simulink model "PWM_Test"  (Simulink 7.7)
settings: Solver=ode4  StartTime=0.0  StopTime=inf  FixedStep=sample_time  RelTol=1e-3
InitFcn:
  | sample_time=0.005;%0.004;%0.0025;%0.02;
  | DeltaT = 0.02;
  | g = 9.81;
  | H0 = g%0.3165;
  | Kl = 1;
  | 
  | Omega_r = 1.6;%for Horizontal reference
  | Zeta_r = 1; %for Horizontal reference
  | Omega = 1.8;%for Horizontal Control
  | Zeta = 0.5;    %for Horizontal Control
  | 
  | Omega_h_r = 2.5; %for vertical reference
  | Zeta_h_r = 0.8;  %for vertical reference
  | Omega_h = 2.7;    %for vertical control
  | Zeta_h = 0.8;         %for vertical control
  | PI=pi;
  | 
  | Mass = 1.15;
  | Acc_Max = 4;
  | Acc_Max_h = 4;
  | 
  | Max_RP = 60;
  | 
  | % for NN
  | n = 5;
  | r = 3;
  | n2 = 5;
  | NN_ST = 0.02;
  | 
  | GAMA_V = 6;
  | gama_V_e = 0.01;
  | 
  | GAMA_W = GAMA_V;
  | gama_W_e =0.01;
  | 
  | % deadzone
  | NN_Deadzone_Z = 0;
  | 
  | % inputs nomalizaton parameters
  | NN_Z_y_min = -3;
  | NN_Z_y_max = 0.5;
  | 
  | NN_Z_v_max = 8;
  | NN_Z_v_min = -NN_Z_v_max;
  | 
  | % alpha = 0.034;
  | alpha = 1;
  | % c_f = 0.0015;
  | c_f = 0.001;
  | c_y_tilt = 1*0.5;
  | 
  | %for WK paras
  | Heightcontrol = 0.08;
  | Scale_Factor=1;
  | yoffset=0;
  | 
  | load MaoBi_Oct04_2_int.mat
  | MB_Interp.time = [];
undefined symbols (not defined in the file or in its folder): DiscIntNeverNeededParam
libraries: simulink x7, dspadpt3 x3, nid_lib x2, X330_Control x2
(part 2 of 2)

== system PWM_Test/Vicon_Data/Filter7 ==
  In1 : Inport
  Kalman Filter : dspadpt3/Kalman Filter  SystemSampleTime=-1  num_targets=1  sourceEnable=Always  isReset=on  X=zeros([12, 1])  P=zeros(12)  A=[1 sample_time sample_time*sample_time/2 zeros(1,9);0 1 sample_time zeros(1,9);0 0 1 zeros(1,9);0 0 0 1 sample_time sample_time*sample_time/2 zeros(1,6);zeros(1,4) 1 sample_time zeros(1,6);zeros(1,5) 1 zeros(1,6);zeros(1,6) 1 sample_time sample_time*sample_time/2 zeros(1,3);zeros(1,7) 1 sample_time zeros(1,3);zeros(1,8) 1 zeros(1,3);zeros(1,9) 1 sample_time sample_time*sample_time/2;zeros(1,10) 1 sample_time;zeros(1,11) 1];  sourceMeasure=Specify via Dialog  H=[1 zeros(1,11); zeros(1,3) 1 zeros(1,8);zeros(1,6) 1 zeros(1,5);zeros(1,9) 1 0 0]  Q=diag([0 0.001 0.001 0 0.001 0.001 0 0.001 0.001 0 0.001 0.001]);  R=diag([0.001 0.001 0.001 0.05])  isOutputEstMeasure=off  isOutputEstState=on  isOutputEstError=off  isOutputPrdMeasure=off  isOutputPrdState=off  isOutputPrdError=off
  Selector1 : Selector  InputPortWidth=12  IndexOptions=Index vector (dialog)  Indices=[10]  OutputSizes=1
  Selector5 : Selector  InputPortWidth=12  IndexOptions=Index vector (dialog)  Indices=[2 5 8]  OutputSizes=1
  Selector6 : Selector  InputPortWidth=12  IndexOptions=Index vector (dialog)  Indices=[3 6 9]  OutputSizes=1
  Vel : Outport
  Acc : Outport  Port=2
  Psi : Outport  Port=3
  wires:
  Selector1/1 -> Psi/1
  Selector5/1 -> Vel/1
  In1/1 -> Kalman Filter/1
  Kalman Filter/1 -> Selector1/1, Selector5/1, Selector6/1
  Selector6/1 -> Acc/1

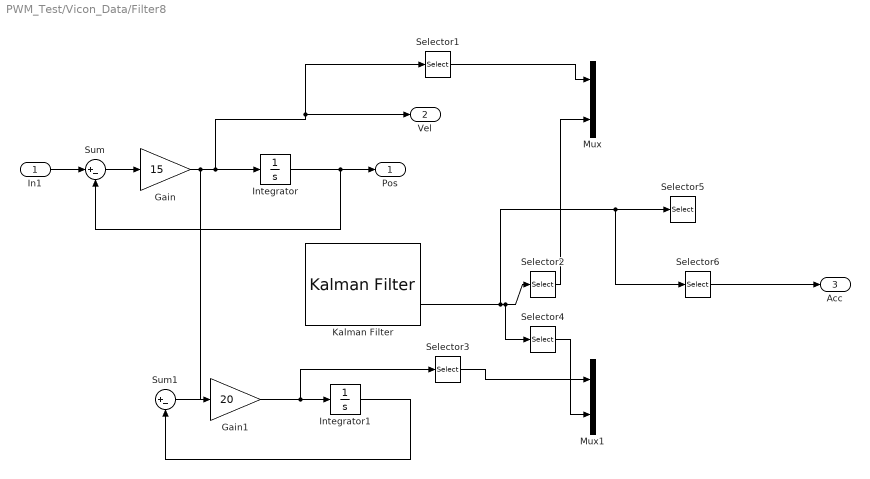
== system PWM_Test/Vicon_Data/Filter8 ==
  In1 : Inport
  Gain : Gain  Gain=15
  Gain1 : Gain  Gain=20
  Integrator : Integrator
  Integrator1 : Integrator
  Kalman Filter : dspadpt3/Kalman Filter  SystemSampleTime=-1  num_targets=1  sourceEnable=Always  isReset=on  X=zeros([9, 1])  P=zeros(9)  A=[1 sample_time sample_time*sample_time/2 zeros(1,6);0 1 sample_time zeros(1,6);0 0 1 zeros(1,6);0 0 0 1 sample_time sample_time*sample_time/2 0 0 0;zeros(1,4) 1 sample_time zeros(1,3);zeros(1,5) 1 zeros(1,3);zeros(1,6) 1 sample_time sample_time*sample_time/2;zeros(1,7) 1 sample_time;zeros(1,8) 1]  sourceMeasure=Specify via Dialog  H=[1 zeros(1,8); zeros(1,3) 1 zeros(1,5);zeros(1,6) 1 0 0]  Q=diag([0 0.001 0.001 0 0.001 0.001 0 0.001 0.001])  R=0.001*eye(3)  isOutputEstMeasure=on  isOutputEstState=on  isOutputEstError=off  isOutputPrdMeasure=off  isOutputPrdState=off  isOutputPrdError=off
  Mux : Mux  Inputs=2
  Mux1 : Mux  Inputs=2
  Selector1 : Selector  InputPortWidth=3  IndexOptions=Index vector (dialog)  Indices=[2]  OutputSizes=1
  Selector2 : Selector  InputPortWidth=9  IndexOptions=Index vector (dialog)  Indices=[5]  OutputSizes=1
  Selector3 : Selector  InputPortWidth=3  IndexOptions=Index vector (dialog)  Indices=[2]  OutputSizes=1
  Selector4 : Selector  InputPortWidth=9  IndexOptions=Index vector (dialog)  Indices=[6]  OutputSizes=1
  Selector5 : Selector  InputPortWidth=9  IndexOptions=Index vector (dialog)  Indices=[2 5 8]  OutputSizes=1
  Selector6 : Selector  InputPortWidth=9  IndexOptions=Index vector (dialog)  Indices=[3 6 9]  OutputSizes=1
  Sum : Sum  Inputs=|+-
  Sum1 : Sum  Inputs=|+-
  Pos : Outport
  Vel : Outport  Port=2
  Acc : Outport  Port=3
  wires:
  Selector6/1 -> Acc/1
  Selector4/1 -> Mux1/2
  Selector3/1 -> Mux1/1
  Selector2/1 -> Mux/2
  Integrator1/1 -> Sum1/2
  Gain1/1 -> Selector3/1, Integrator1/1
  Sum1/1 -> Gain1/1
  Kalman Filter/2 -> Selector6/1, Selector5/1, Selector2/1, Selector4/1
  Selector1/1 -> Mux/1
  In1/1 -> Sum/1
  Integrator/1 -> Sum/2, Pos/1
  Gain/1 -> Sum1/1, Vel/1, Selector1/1, Integrator/1
  Sum/1 -> Gain/1

== system PWM_Test/Vicon_Data/Raw Quad Pose from Vicon ==
  Constant : Constant
  Demux : Demux  Outputs=3
  Interpreted MATLAB Function : MATLABFcn  MATLABFcn=JXKinect05112013
  Process Vicon Raw Data1 : Subsystem
  Process Vicon Raw Data6 : Subsystem
  Process Vicon Raw Data7 : Subsystem
  Position_Vicon_JianXing : Outport
  Attitude_Vicon_JianXing : Outport  Port=2
  Position_Vicon_K platform : Outport  Port=3
  Attitude_Vicon_K platform : Outport  Port=4
  Position_Vicon_draw : Outport  Port=5
  Attitude_Vicon_draw : Outport  Port=6
  wires:
  Demux/3 -> Process Vicon Raw Data1/1(Vicon Raw)
  Process Vicon Raw Data1/1(Position) -> Position_Vicon_draw/1
  Process Vicon Raw Data1/2(Attitude) -> Attitude_Vicon_draw/1
  Demux/2 -> Process Vicon Raw Data7/1(Vicon Raw)
  Process Vicon Raw Data7/1(Position) -> Position_Vicon_K platform/1
  Process Vicon Raw Data7/2(Attitude) -> Attitude_Vicon_K platform/1
  Constant/1 -> Interpreted MATLAB Function/1
  Demux/1 -> Process Vicon Raw Data6/1(Vicon Raw)
  Process Vicon Raw Data6/1(Position) -> Position_Vicon_JianXing/1
  Process Vicon Raw Data6/2(Attitude) -> Attitude_Vicon_JianXing/1
  Interpreted MATLAB Function/1 -> Demux/1

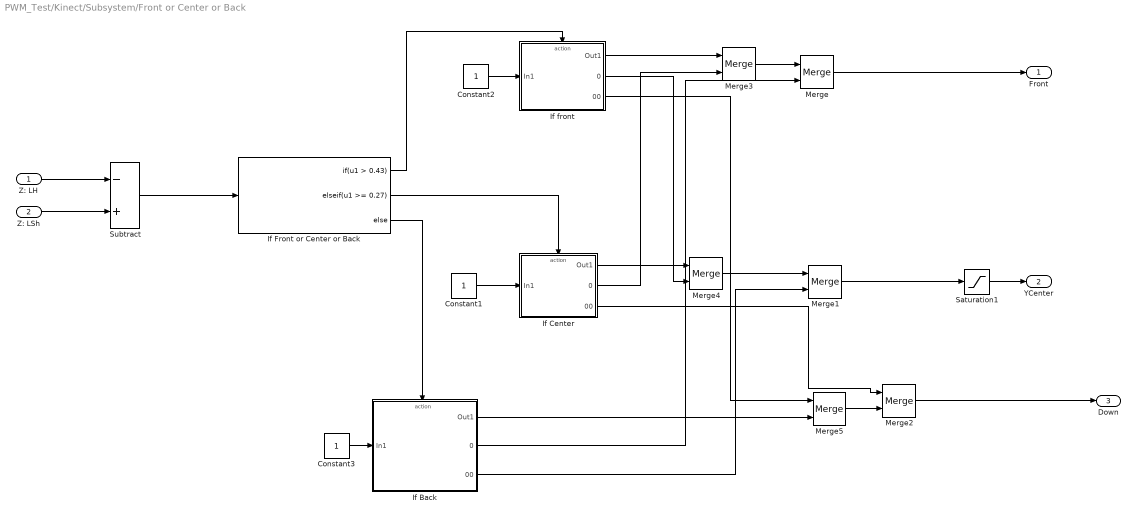
== system PWM_Test/Kinect/Subsystem/Front or Center or Back ==
  Z: LH : Inport
  Z: LSh : Inport  Port=2
  Constant1 : Constant
  Constant2 : Constant
  Constant3 : Constant
  If Back : Subsystem  TreatAsAtomicUnit=on
  If Center : Subsystem  TreatAsAtomicUnit=on
  If Front or Center or Back : If  IfExpression=u1 > 0.43  ElseIfExpressions=u1 >= 0.27
  If front : Subsystem  TreatAsAtomicUnit=on
  Merge{,1..5} (6 alike) : Merge
  Saturation1 : Saturate  UpperLimit=1  LowerLimit=0
  Subtract : Sum  Inputs=-+
  Front : Outport
  YCenter : Outport  Port=2
  Down : Outport  Port=3
  wires:
  Z: LH/1 -> Subtract/1
  Z: LSh/1 -> Subtract/2
  Subtract/1 -> If Front or Center or Back/1
  If Front or Center or Back/1 -> If front/Action
  If Front or Center or Back/2 -> If Center/Action
  If Front or Center or Back/3 -> If Back/Action
  Merge3/1 -> Merge/1
  Merge4/1 -> Merge1/1
  If front/1(Out1) -> Merge3/1
  If Center/1(Out1) -> Merge4/1
  Merge5/1 -> Merge2/2
  If Back/1(Out1) -> Merge5/2
  If front/2(0) -> Merge4/2
  If front/3(00) -> Merge5/1
  If Center/2(0) -> Merge3/2
  If Back/2(0) -> Merge/2
  If Center/3(00) -> Merge2/1
  If Back/3(00) -> Merge1/2
  Merge1/1 -> Saturation1/1
  Saturation1/1 -> YCenter/1
  Constant2/1 -> If front/1(In1)
  Merge/1 -> Front/1
  Constant1/1 -> If Center/1(In1)
  Constant3/1 -> If Back/1(In1)
  Merge2/1 -> Down/1

== system PWM_Test/Kinect/Subsystem/Left or Center or Right ==
  X: LH : Inport
  X: LSh : Inport  Port=2
  If Action Subsystem : Subsystem  TreatAsAtomicUnit=on
  If Action Subsystem1 : Subsystem  TreatAsAtomicUnit=on
  If Left or Right : If  NumInputs=2  IfExpression=u1 >= u2
  Merge{,1..3} (4 alike) : Merge  InitialOutput=[0]
  Saturation : Saturate  UpperLimit=1  LowerLimit=0
  Sum of Elements : Sum  Inputs=+|+
  Left : Outport
  X Center : Outport  Port=2
  Right : Outport  Port=3
  wires:
  X: LH/1 -> If Action Subsystem/1(x:LH), If Left or Right/1, If Action Subsystem1/1(x: LH)
  X: LSh/1 -> If Action Subsystem/2(x:LSh), If Left or Right/2, If Action Subsystem1/2(x: LSh)
  Saturation/1 -> X Center/1
  If Left or Right/2 -> If Action Subsystem1/Action
  If Left or Right/1 -> If Action Subsystem/Action
  Merge1/1 -> Sum of Elements/1
  Merge2/1 -> Sum of Elements/2
  If Action Subsystem1/1(Center) -> Merge2/2
  Merge3/1 -> Right/1
  If Action Subsystem1/2(Right) -> Merge3/2
  If Action Subsystem/2(Center) -> Merge1/1
  If Action Subsystem/1(Left) -> Merge/1
  If Action Subsystem/3(0) -> Merge3/1
  If Action Subsystem1/3(0) -> Merge/2
  If Action Subsystem/4(00) -> Merge2/1
  If Action Subsystem1/4(00) -> Merge1/2
  Merge/1 -> Left/1
  Sum of Elements/1 -> Saturation/1

== system PWM_Test/Kinect/Subsystem/Up or Center or Down ==
  Y: LH : Inport
  Y: LSh : Inport  Port=2
  If Down or Center : Subsystem  TreatAsAtomicUnit=on
  If Left or Right : If  NumInputs=2  IfExpression=u1 >= u2
  If Up or Center : Subsystem  TreatAsAtomicUnit=on
  Merge{,1..3} (4 alike) : Merge
  Saturation : Saturate  UpperLimit=1  LowerLimit=0
  Sum of Elements : Sum  Inputs=+|+
  Top : Outport
  ZCenter : Outport  Port=2
  Down : Outport  Port=3
  wires:
  If Left or Right/2 -> If Down or Center/Action
  If Left or Right/1 -> If Up or Center/Action
  Y: LH/1 -> If Left or Right/1, If Up or Center/1(Y: LH), If Down or Center/1(Y: LH)
  Y: LSh/1 -> If Left or Right/2, If Up or Center/2(Y: LSh), If Down or Center/2(Y: LSh)
  Saturation/1 -> ZCenter/1
  Merge/1 -> Top/1
  If Up or Center/1(Top) -> Merge/1
  Merge1/1 -> Down/1
  If Down or Center/2(Down) -> Merge1/1
  If Down or Center/3(0) -> Merge/2
  If Up or Center/3(0) -> Merge1/2
  If Up or Center/2(Center) -> Merge2/1
  If Down or Center/1(Center) -> Merge3/2
  If Up or Center/4(00) -> Merge3/1
  If Down or Center/4(00) -> Merge2/2
  Merge2/1 -> Sum of Elements/1
  Merge3/1 -> Sum of Elements/2
  Sum of Elements/1 -> Saturation/1

== system PWM_Test/Kinect/Subsystem1/Left or Center or Right ==
  X: RH : Inport
  X: RSh : Inport  Port=2
  If Left or Right : If  NumInputs=2  IfExpression=u1 >= u2
  Left or Center : Subsystem  TreatAsAtomicUnit=on
  Merge{,1..3} (4 alike) : Merge  InitialOutput=[0]
  Right or Center : Subsystem  TreatAsAtomicUnit=on
  Saturation : Saturate  UpperLimit=1  LowerLimit=0
  Sum of Elements : Sum  Inputs=+|+
  Left : Outport
  X Center : Outport  Port=2
  Right : Outport  Port=3
  wires:
  X: RH/1 -> Left or Center/1(x:RH), If Left or Right/1, Right or Center/1(x: RH)
  X: RSh/1 -> Left or Center/2(x:RSh), If Left or Right/2, Right or Center/2(x: RSh)
  Sum of Elements/1 -> Saturation/1
  Saturation/1 -> X Center/1
  If Left or Right/2 -> Right or Center/Action
  Merge1/1 -> Sum of Elements/1
  Merge2/1 -> Sum of Elements/2
  Right or Center/1(Center) -> Merge2/2
  Right or Center/2(Right) -> Merge3/2
  Left or Center/2(Center) -> Merge1/1
  Left or Center/1(Left) -> Merge/1
  Left or Center/3(0) -> Merge3/1
  Right or Center/3(0) -> Merge/2
  Left or Center/4(00) -> Merge2/1
  Right or Center/4(00) -> Merge1/2
  If Left or Right/1 -> Left or Center/Action
  Merge/1 -> Left/1
  Merge3/1 -> Right/1

== system PWM_Test/Kinect/Subsystem1/Up or Center or Down ==
  Y: RH : Inport
  Y: RSh : Inport  Port=2
  If Down or Center : Subsystem  TreatAsAtomicUnit=on
  If Left or Right : If  NumInputs=2  IfExpression=u1 >= u2
  If Up or Center : Subsystem  TreatAsAtomicUnit=on
  Merge{,1..3} (4 alike) : Merge
  Saturation : Saturate  UpperLimit=1  LowerLimit=0
  Sum of Elements : Sum  Inputs=+|+
  Top : Outport
  ZCenter : Outport  Port=2
  Down : Outport  Port=3
  wires:
  If Left or Right/2 -> If Down or Center/Action
  If Left or Right/1 -> If Up or Center/Action
  Y: RH/1 -> If Left or Right/1, If Up or Center/1(Y: RH), If Down or Center/1(Y: RH)
  Y: RSh/1 -> If Left or Right/2, If Up or Center/2(Y: RSh), If Down or Center/2(Y: RSh)
  Sum of Elements/1 -> Saturation/1
  Saturation/1 -> ZCenter/1
  Merge/1 -> Top/1
  If Up or Center/1(Top) -> Merge/1
  Merge1/1 -> Down/1
  If Down or Center/2(Down) -> Merge1/1
  If Down or Center/3(0) -> Merge/2
  If Up or Center/3(0) -> Merge1/2
  If Up or Center/2(Center) -> Merge2/1
  If Down or Center/1(Center) -> Merge3/2
  If Up or Center/4(00) -> Merge3/1
  If Down or Center/4(00) -> Merge2/2
  Merge2/1 -> Sum of Elements/1
  Merge3/1 -> Sum of Elements/2

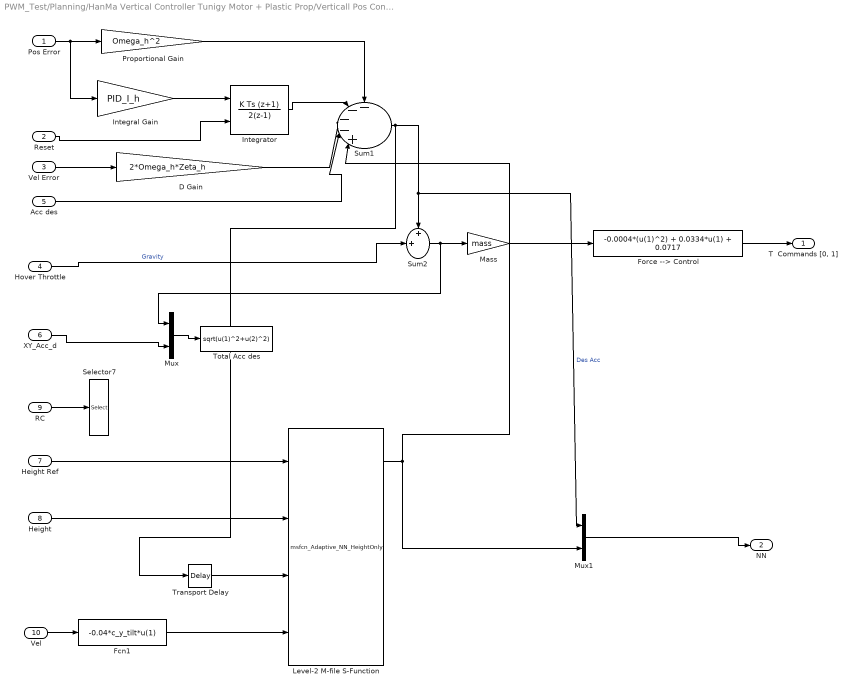
== system PWM_Test/Planning/HanMa Vertical Controller Tunigy Motor + Plastic Prop/Verticall Pos Controller ==
  Pos Error : Inport
  Reset : Inport  Port=2
  Vel Error : Inport  Port=3
  Hover Throttle : Inport  Port=4
  Acc des : Inport  Port=5
  XY_Acc_d : Inport  Port=6
  Height Ref : Inport  Port=7
  Height : Inport  Port=8
  RC : Inport  Port=9
  Vel : Inport  Port=10
  D Gain : Gain  Gain=2*Omega_h*Zeta_h  OutDataTypeStr=double
  Fcn1 : Fcn  Expr=-0.04*c_y_tilt*u(1)
  Force --> Control : Fcn  Expr=-0.0004*(u(1)^2) + 0.0334*u(1) + 0.0717
  Integral Gain : Gain  DisableCoverage=on  Gain=PID_I_h  ParamDataTypeStr=double  OutDataTypeStr=double
  Integrator : DiscreteIntegrator  DisableCoverage=on  IntegratorMethod=Integration: Trapezoidal  ExternalReset=rising  InitialConditionMode=State only (most efficient)  SampleTime=-1  OutDataTypeStr=double  UpperSaturationLimit=0.3  LowerSaturationLimit=-0.3  ICPrevOutput=DiscIntNeverNeededParam  ICPrevScaledInput=DiscIntNeverNeededParam
  Level-2 M-file S-Function : M-S-Function  FunctionName=msfcn_Adaptive_NN_HeightOnly  Parameters=n,r,n2,NN_ST,GAMA_V,gama_V_e,GAMA_W,gama_W_e,alpha,c_f,c_y_tilt,NN_Deadzone_Z,NN_Z_y_min,NN_Z_y_max,NN_Z_v_min,NN_Z_v_max
      mask Display: fprintf('Output Feedback NN \n Control Block')
  Mass : Gain  DisableCoverage=on  Gain=mass  ParamDataTypeStr=double  OutDataTypeStr=double
  Mux : Mux  Inputs=2
  Mux1 : Mux  Inputs=2
  Proportional Gain : Gain  DisableCoverage=on  Gain=Omega_h^2  ParamDataTypeStr=double  OutDataTypeStr=double
  Selector7 : Selector  InputPortWidth=8  IndexOptions=Index vector (dialog)  Indices=[6]  OutputSizes=1
  Sum1 : Sum  DisableCoverage=on  Inputs=----+|  AccumDataTypeStr=double  OutDataTypeStr=double  SampleTime=0.02
  Sum2 : Sum  DisableCoverage=on  Inputs=++|  AccumDataTypeStr=double  OutDataTypeStr=double  SampleTime=0.02
  Total Acc des : Fcn  Expr=sqrt(u(1)^2+u(2)^2)
  Transport Delay : TransportDelay  DelayTime=0.02
  "T  Commands [0, 1]" : Outport
  NN : Outport  Port=2
  wires:
  Force --> Control/1 -> "T  Commands [0, 1]"/1
  Sum2/1 -> Mux/1, Mass/1
  XY_Acc_d/1 -> Mux/2
  Mux/1 -> Total Acc des/1
  Mass/1 -> Force --> Control/1
  Sum1/1 -> Transport Delay/1, Sum2/1, Mux1/1  "Des Acc"
  Hover Throttle/1 -> Sum2/2  "Gravity"
  Acc des/1 -> Sum1/4
  D Gain/1 -> Sum1/3
  Vel Error/1 -> D Gain/1
  Reset/1 -> Integrator/2
  Pos Error/1 -> Integral Gain/1, Proportional Gain/1
  Proportional Gain/1 -> Sum1/1
  Integrator/1 -> Sum1/2
  Integral Gain/1 -> Integrator/1
  Height Ref/1 -> Level-2 M-file S-Function/1
  Level-2 M-file S-Function/1 -> Mux1/2, Sum1/5
  RC/1 -> Selector7/1
  Fcn1/1 -> Level-2 M-file S-Function/4
  Transport Delay/1 -> Level-2 M-file S-Function/3
  Mux1/1 -> NN/1
  Vel/1 -> Fcn1/1
  Height/1 -> Level-2 M-file S-Function/2

== system PWM_Test/Planning/Yaw Controller/Heading ==
  u : Inport  SampleTime=SampleTime
  RESET : Inport  Port=2  SampleTime=SampleTime
  Integral Gain : Gain  DisableCoverage=on  Gain=I  ParamMin=IParamMin  ParamMax=IParamMax  ParamDataTypeStr=IParamDataTypeStr  OutMin=IOutMin  OutMax=IOutMax  OutDataTypeStr=IOutDataTypeStr
  Integrator : DiscreteIntegrator  DisableCoverage=on  IntegratorMethod=Integration: Trapezoidal  ExternalReset=rising  InitialCondition=InitialConditionForIntegrator  InitialConditionMode=State only (most efficient)  SampleTime=-1  OutMin=IntegratorOutMin  OutMax=IntegratorOutMax  OutDataTypeStr=IntegratorOutDataTypeStr  ICPrevOutput=DiscIntNeverNeededParam  ICPrevScaledInput=DiscIntNeverNeededParam
  Proportional Gain : Gain  DisableCoverage=on  Gain=P  ParamMin=PParamMin  ParamMax=PParamMax  ParamDataTypeStr=PParamDataTypeStr  OutMin=POutMin  OutMax=POutMax  OutDataTypeStr=POutDataTypeStr
  Saturation : Saturate  UpperLimit=UpperSaturationLimit  LowerLimit=LowerSaturationLimit  LinearizeAsGain=off  OutMin=SaturationOutMin  OutMax=SaturationOutMax  OutDataTypeStr=SaturationOutDataTypeStr
  Sum : Sum  DisableCoverage=on  Inputs=++|  AccumDataTypeStr=SumAccumDataTypeStr  OutMin=SumOutMin  OutMax=SumOutMax  OutDataTypeStr=SumOutDataTypeStr
  y : Outport  InitialOutput=0
  wires:
  Sum/1 -> Saturation/1
  Saturation/1 -> y/1
  RESET/1 -> Integrator/2
  Proportional Gain/1 -> Sum/1
  Integrator/1 -> Sum/2
  Integral Gain/1 -> Integrator/1
  u/1 -> Proportional Gain/1, Integral Gain/1

== system PWM_Test/Vicon_Data/Raw Quad Pose from Vicon/Process Vicon Raw Data1 ==
  note: Z
  note: Y
  note: X
  Vicon Raw : Inport
  Add1 : Sum  Inputs=-+
  Constant1 : Constant  Value=pi  OutDataTypeStr=double
  Demux : Demux  Outputs=6
  Flip_pi1 : Subsystem
      mask Type: Flip -pi to pi
      mask Description: Flips the inputs into the range -pi to pi
      mask Help: Flips the inputs into the range -pi to pi
      mask Display: disp('Flip_pi')
  Gain1 : Gain  Gain=0.001
  Gain3 : Gain  Gain=-1
  Gain6 : Gain  Gain=-0.001
  Gain7 : Gain  Gain=-0.001
  Matrix Concatenate1 : Concatenate  NumInputs=3  Mode=Multidimensional array
  Matrix Concatenate13 : Concatenate  NumInputs=3  Mode=Multidimensional array
  Position : Outport
  Attitude : Outport  Port=2
  wires:
  Matrix Concatenate1/1 -> Attitude/1
  Vicon Raw/1 -> Demux/1
  Matrix Concatenate13/1 -> Position/1
  Flip_pi1/1(Angle_Flip) -> Matrix Concatenate1/1
  Demux/5 -> Matrix Concatenate1/2  "pitch"
  Gain3/1 -> Flip_pi1/1(Angle)
  Add1/1 -> Gain3/1
  Gain7/1 -> Matrix Concatenate13/3
  Gain6/1 -> Matrix Concatenate13/2
  Demux/4 -> Add1/1  "roll"
  Demux/3 -> Gain7/1
  Demux/2 -> Gain6/1
  Demux/1 -> Gain1/1
  Gain1/1 -> Matrix Concatenate13/1
  Demux/6 -> Matrix Concatenate1/3  "yaw"
  Constant1/1 -> Add1/2

== system PWM_Test/Vicon_Data/Raw Quad Pose from Vicon/Process Vicon Raw Data6 ==
  note: Z
  note: Y
  note: X
  Vicon Raw : Inport
  Add1 : Sum  Inputs=-+
  Constant1 : Constant  Value=pi  OutDataTypeStr=double
  Demux : Demux  Outputs=6
  Flip_pi1 : Subsystem
      mask Type: Flip -pi to pi
      mask Description: Flips the inputs into the range -pi to pi
      mask Help: Flips the inputs into the range -pi to pi
      mask Display: disp('Flip_pi')
  Gain1 : Gain  Gain=0.001
  Gain3 : Gain  Gain=-1
  Gain6 : Gain  Gain=-0.001
  Gain7 : Gain  Gain=-0.001
  Matrix Concatenate1 : Concatenate  NumInputs=3  Mode=Multidimensional array
  Matrix Concatenate13 : Concatenate  NumInputs=3  Mode=Multidimensional array
  Position : Outport
  Attitude : Outport  Port=2
  wires:
  Matrix Concatenate1/1 -> Attitude/1
  Vicon Raw/1 -> Demux/1
  Matrix Concatenate13/1 -> Position/1
  Flip_pi1/1(Angle_Flip) -> Matrix Concatenate1/1
  Demux/5 -> Matrix Concatenate1/2  "pitch"
  Gain3/1 -> Flip_pi1/1(Angle)
  Add1/1 -> Gain3/1
  Gain7/1 -> Matrix Concatenate13/3
  Gain6/1 -> Matrix Concatenate13/2
  Demux/4 -> Add1/1  "roll"
  Demux/3 -> Gain7/1
  Demux/2 -> Gain6/1
  Demux/1 -> Gain1/1
  Gain1/1 -> Matrix Concatenate13/1
  Demux/6 -> Matrix Concatenate1/3  "yaw"
  Constant1/1 -> Add1/2

== system PWM_Test/Vicon_Data/Raw Quad Pose from Vicon/Process Vicon Raw Data7 ==
  note: X
  note: Y
  note: Z
  Vicon Raw : Inport
  Add1 : Sum  Inputs=-+
  Constant1 : Constant  Value=pi  OutDataTypeStr=double
  Demux : Demux  Outputs=6
  Flip_pi1 : Subsystem
      mask Type: Flip -pi to pi
      mask Description: Flips the inputs into the range -pi to pi
      mask Help: Flips the inputs into the range -pi to pi
      mask Display: disp('Flip_pi')
  Gain1 : Gain  Gain=0.001
  Gain3 : Gain  Gain=-1
  Gain6 : Gain  Gain=-0.001
  Gain7 : Gain  Gain=-0.001
  Matrix Concatenate1 : Concatenate  NumInputs=3  Mode=Multidimensional array
  Matrix Concatenate13 : Concatenate  NumInputs=3  Mode=Multidimensional array
  Position : Outport
  Attitude : Outport  Port=2
  wires:
  Constant1/1 -> Add1/2
  Demux/6 -> Matrix Concatenate1/3  "yaw"
  Gain1/1 -> Matrix Concatenate13/1
  Demux/1 -> Gain1/1
  Demux/2 -> Gain6/1
  Demux/3 -> Gain7/1
  Demux/4 -> Add1/1  "roll"
  Gain6/1 -> Matrix Concatenate13/2
  Gain7/1 -> Matrix Concatenate13/3
  Add1/1 -> Gain3/1
  Gain3/1 -> Flip_pi1/1(Angle)
  Demux/5 -> Matrix Concatenate1/2  "pitch"
  Flip_pi1/1(Angle_Flip) -> Matrix Concatenate1/1
  Matrix Concatenate13/1 -> Position/1
  Vicon Raw/1 -> Demux/1
  Matrix Concatenate1/1 -> Attitude/1

== system PWM_Test/Kinect/Subsystem/Front or Center or Back/If Back ==
  In1 : Inport
  Action Port : ActionPort  ActionType=else
  Constant : Constant  Value=0
  Constant1 : Constant  Value=0
  Out1 : Outport
  0 : Outport  Port=2
  00 : Outport  Port=3
  wires:
  In1/1 -> Out1/1
  Constant/1 -> 0/1
  Constant1/1 -> 00/1

== system PWM_Test/Kinect/Subsystem/Front or Center or Back/If Center ==
  In1 : Inport
  Action Port : ActionPort  ActionType=elseif
  Constant : Constant  Value=0
  Constant1 : Constant  Value=0
  Out1 : Outport
  0 : Outport  Port=2
  00 : Outport  Port=3
  wires:
  In1/1 -> Out1/1
  Constant/1 -> 0/1
  Constant1/1 -> 00/1

== system PWM_Test/Kinect/Subsystem/Front or Center or Back/If front ==
  In1 : Inport
  Action Port : ActionPort  ActionType=then
  Constant : Constant  Value=0
  Constant1 : Constant  Value=0
  Out1 : Outport
  0 : Outport  Port=2
  00 : Outport  Port=3
  wires:
  In1/1 -> Out1/1
  Constant/1 -> 0/1
  Constant1/1 -> 00/1

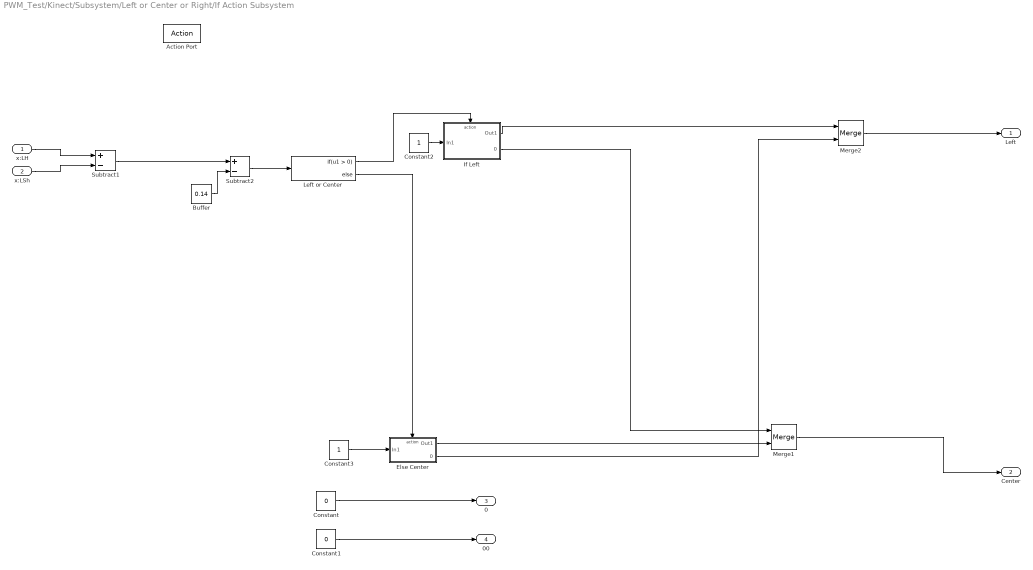
== system PWM_Test/Kinect/Subsystem/Left or Center or Right/If Action Subsystem ==
  x:LH : Inport
  x:LSh : Inport  Port=2
  Action Port : ActionPort  InitializeStates=reset  ActionType=then
  Buffer : Constant  Value=0.14
  Constant : Constant  Value=0
  Constant1 : Constant  Value=0
  Constant2 : Constant
  Constant3 : Constant
  Else Center : Subsystem  TreatAsAtomicUnit=on
  If Left : Subsystem  TreatAsAtomicUnit=on
  Left or Center : If
  Merge1 : Merge  InitialOutput=[0]
  Merge2 : Merge  InitialOutput=[0]
  Subtract1 : Sum  Inputs=+-
  Subtract2 : Sum  Inputs=+-
  Left : Outport
  Center : Outport  Port=2
  0 : Outport  Port=3
  00 : Outport  Port=4
  wires:
  Buffer/1 -> Subtract2/2
  Subtract2/1 -> Left or Center/1
  x:LH/1 -> Subtract1/1
  x:LSh/1 -> Subtract1/2
  Subtract1/1 -> Subtract2/1
  Merge2/1 -> Left/1
  Merge1/1 -> Center/1
  Else Center/1(Out1) -> Merge1/2
  If Left/1(Out1) -> Merge2/1
  Left or Center/1 -> If Left/Action
  Left or Center/2 -> Else Center/Action
  If Left/2(0) -> Merge1/1
  Else Center/2(0) -> Merge2/2
  Constant/1 -> 0/1
  Constant1/1 -> 00/1
  Constant2/1 -> If Left/1(In1)
  Constant3/1 -> Else Center/1(In1)

== system PWM_Test/Kinect/Subsystem/Left or Center or Right/If Action Subsystem1 ==
  x: LH : Inport
  x: LSh : Inport  Port=2
  Action Port : ActionPort  InitializeStates=reset  ActionType=else
  Buffer : Constant  Value=0.14
  Constant : Constant  Value=0
  Constant1 : Constant  Value=0
  Constant2 : Constant
  Constant3 : Constant
  Else Hover : Subsystem  TreatAsAtomicUnit=on
  If : If
  If Right : Subsystem  TreatAsAtomicUnit=on
  Merge : Merge  InitialOutput=[0]
  Merge1 : Merge  InitialOutput=[0]
  Subtract1 : Sum  Inputs=+-
  Subtract2 : Sum  Inputs=+-
  Center : Outport
  Right : Outport  Port=2
  0 : Outport  Port=3
  00 : Outport  Port=4
  wires:
  Buffer/1 -> Subtract2/2
  Subtract2/1 -> If/1
  If/1 -> If Right/Action
  If/2 -> Else Hover/Action
  x: LSh/1 -> Subtract1/1
  x: LH/1 -> Subtract1/2
  Subtract1/1 -> Subtract2/1
  If Right/1(Out1) -> Merge/1
  Merge1/1 -> Center/1
  Else Hover/1(Out1) -> Merge1/1
  Else Hover/2(0) -> Merge/2
  If Right/2(0) -> Merge1/2
  Merge/1 -> Right/1
  Constant/1 -> 0/1
  Constant1/1 -> 00/1
  Constant2/1 -> If Right/1(In1)
  Constant3/1 -> Else Hover/1(In1)

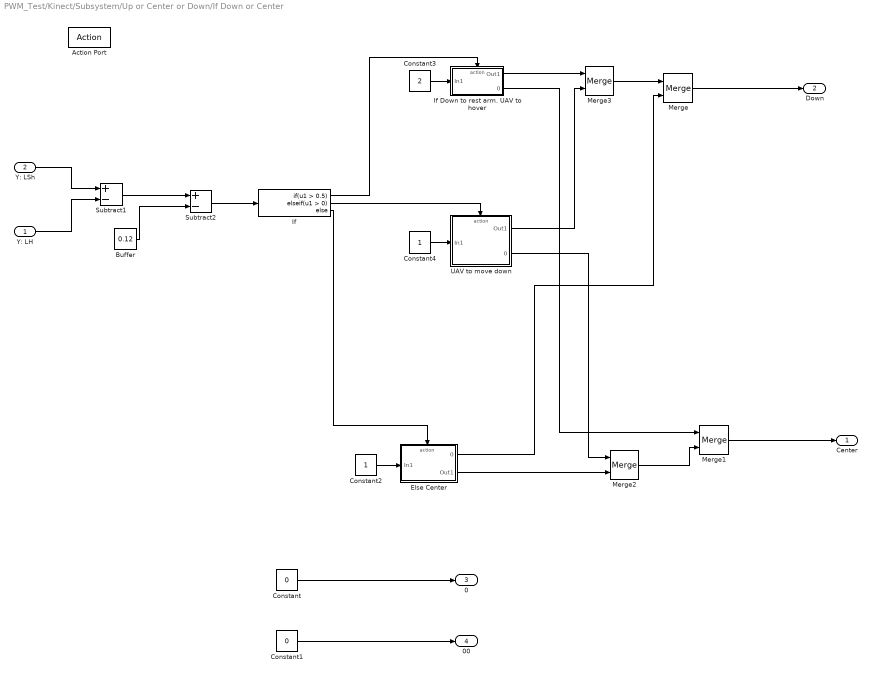
== system PWM_Test/Kinect/Subsystem/Up or Center or Down/If Down or Center ==
  Y: LH : Inport
  Y: LSh : Inport  Port=2
  Action Port : ActionPort  ActionType=else
  Buffer : Constant  Value=0.12
  Constant : Constant  Value=0
  Constant1 : Constant  Value=0
  Constant2 : Constant
  Constant3 : Constant  Value=2
  Constant4 : Constant
  Else Center : Subsystem  TreatAsAtomicUnit=on
  If : If  IfExpression=u1 > 0.5  ElseIfExpressions=u1 > 0
  If Down to rest arm. UAV to hover : Subsystem  TreatAsAtomicUnit=on
  Merge{,1..3} (4 alike) : Merge  InitialOutput=[0]
  Subtract1 : Sum  Inputs=+-
  Subtract2 : Sum  Inputs=+-
  UAV to move down : Subsystem  TreatAsAtomicUnit=on
  Center : Outport
  Down : Outport  Port=2
  0 : Outport  Port=3
  00 : Outport  Port=4
  wires:
  Buffer/1 -> Subtract2/2
  Subtract2/1 -> If/1
  If/1 -> If Down to rest arm. UAV to hover/Action
  If/3 -> Else Center/Action
  Y: LSh/1 -> Subtract1/1
  Y: LH/1 -> Subtract1/2
  Subtract1/1 -> Subtract2/1
  Merge/1 -> Down/1
  Else Center/1(0) -> Merge/2
  Merge1/1 -> Center/1
  If Down to rest arm. UAV to hover/2(0) -> Merge1/1
  Constant/1 -> 0/1
  Constant1/1 -> 00/1
  Constant2/1 -> Else Center/1(In1)
  Constant3/1 -> If Down to rest arm. UAV to hover/1(In1)
  If/2 -> UAV to move down/Action
  Constant4/1 -> UAV to move down/1(In1)
  Else Center/2(Out1) -> Merge2/2
  Merge2/1 -> Merge1/2
  UAV to move down/2(0) -> Merge2/1
  If Down to rest arm. UAV to hover/1(Out1) -> Merge3/1
  Merge3/1 -> Merge/1
  UAV to move down/1(Out1) -> Merge3/2

== system PWM_Test/Kinect/Subsystem/Up or Center or Down/If Up or Center ==
  Y: LH : Inport
  Y: LSh : Inport  Port=2
  Action Port : ActionPort  ActionType=then
  Buffer : Constant  Value=0.12
  Constant : Constant  Value=0
  Constant1 : Constant  Value=0
  Constant2 : Constant
  Constant3 : Constant
  Else Center : Subsystem  TreatAsAtomicUnit=on
  If : If
  If Top : Subsystem  TreatAsAtomicUnit=on
  Merge : Merge  InitialOutput=[0]
  Merge1 : Merge  InitialOutput=[0]
  Subtract1 : Sum  Inputs=+-
  Subtract2 : Sum  Inputs=+-
  Top : Outport
  Center : Outport  Port=2
  0 : Outport  Port=3
  00 : Outport  Port=4
  wires:
  Buffer/1 -> Subtract2/2
  Subtract2/1 -> If/1
  If/1 -> If Top/Action
  If/2 -> Else Center/Action
  Y: LH/1 -> Subtract1/1
  Y: LSh/1 -> Subtract1/2
  Subtract1/1 -> Subtract2/1
  If Top/1(Out1) -> Merge/1
  Else Center/1(0) -> Merge/2
  Merge/1 -> Top/1
  Merge1/1 -> Center/1
  If Top/2(0) -> Merge1/1
  Else Center/2(Out1) -> Merge1/2
  Constant/1 -> 0/1
  Constant1/1 -> 00/1
  Constant2/1 -> If Top/1(In1)
  Constant3/1 -> Else Center/1(In1)

== system PWM_Test/Kinect/Subsystem1/Left or Center or Right/Left or Center ==
  x:RH : Inport
  x:RSh : Inport  Port=2
  Action Port : ActionPort  InitializeStates=reset  ActionType=then
  Buffer : Constant  Value=0.14
  Constant : Constant  Value=0
  Constant1 : Constant  Value=0
  Constant2 : Constant
  Constant3 : Constant
  Else Center : Subsystem  TreatAsAtomicUnit=on
  If : If
  If Left : Subsystem  TreatAsAtomicUnit=on
  Merge1 : Merge  InitialOutput=[0]
  Merge2 : Merge  InitialOutput=[0]
  Subtract1 : Sum  Inputs=+-
  Subtract2 : Sum  Inputs=+-
  Left : Outport
  Center : Outport  Port=2
  0 : Outport  Port=3
  00 : Outport  Port=4
  wires:
  Buffer/1 -> Subtract2/2
  Subtract2/1 -> If/1
  x:RH/1 -> Subtract1/1
  x:RSh/1 -> Subtract1/2
  Subtract1/1 -> Subtract2/1
  Merge2/1 -> Left/1
  Merge1/1 -> Center/1
  Else Center/1(Out1) -> Merge1/2
  If Left/1(Out1) -> Merge2/1
  If/1 -> If Left/Action
  If/2 -> Else Center/Action
  If Left/2(0) -> Merge1/1
  Else Center/2(0) -> Merge2/2
  Constant/1 -> 0/1
  Constant1/1 -> 00/1
  Constant2/1 -> If Left/1(In1)
  Constant3/1 -> Else Center/1(In1)

== system PWM_Test/Kinect/Subsystem1/Left or Center or Right/Right or Center ==
  x: RH : Inport
  x: RSh : Inport  Port=2
  Action Port : ActionPort  InitializeStates=reset  ActionType=else
  Buffer : Constant  Value=0.14
  Constant : Constant  Value=0
  Constant1 : Constant  Value=0
  Constant2 : Constant
  Constant3 : Constant
  Else Center : Subsystem  TreatAsAtomicUnit=on
  If : If
  If Right : Subsystem  TreatAsAtomicUnit=on
  Merge : Merge  InitialOutput=[0]
  Merge1 : Merge  InitialOutput=[0]
  Subtract1 : Sum  Inputs=+-
  Subtract2 : Sum  Inputs=+-
  Center : Outport
  Right : Outport  Port=2
  0 : Outport  Port=3
  00 : Outport  Port=4
  wires:
  Buffer/1 -> Subtract2/2
  Subtract2/1 -> If/1
  If/1 -> If Right/Action
  If/2 -> Else Center/Action
  x: RSh/1 -> Subtract1/1
  x: RH/1 -> Subtract1/2
  Subtract1/1 -> Subtract2/1
  If Right/1(Out1) -> Merge/1
  Merge1/1 -> Center/1
  Else Center/1(Out1) -> Merge1/1
  Else Center/2(0) -> Merge/2
  If Right/2(0) -> Merge1/2
  Merge/1 -> Right/1
  Constant/1 -> 0/1
  Constant1/1 -> 00/1
  Constant2/1 -> If Right/1(In1)
  Constant3/1 -> Else Center/1(In1)

== system PWM_Test/Kinect/Subsystem1/Up or Center or Down/If Down or Center ==
  Y: RH : Inport
  Y: RSh : Inport  Port=2
  Action Port : ActionPort  ActionType=else
  Buffer : Constant  Value=0.14
  Constant : Constant  Value=0
  Constant1 : Constant  Value=0
  Constant2 : Constant
  Constant3 : Constant
  Else Center : Subsystem  TreatAsAtomicUnit=on
  If : If
  If Down to rest arm. UAV to hover : Subsystem  TreatAsAtomicUnit=on
  Merge : Merge  InitialOutput=[0]
  Merge1 : Merge  InitialOutput=[0]
  Subtract1 : Sum  Inputs=+-
  Subtract2 : Sum  Inputs=+-
  Center : Outport
  Down : Outport  Port=2
  0 : Outport  Port=3
  00 : Outport  Port=4
  wires:
  Buffer/1 -> Subtract2/2
  Subtract2/1 -> If/1
  If/1 -> If Down to rest arm. UAV to hover/Action
  If/2 -> Else Center/Action
  Y: RSh/1 -> Subtract1/1
  Y: RH/1 -> Subtract1/2
  Subtract1/1 -> Subtract2/1
  Merge/1 -> Down/1
  Else Center/1(0) -> Merge/2
  Merge1/1 -> Center/1
  If Down to rest arm. UAV to hover/2(0) -> Merge1/1
  Constant/1 -> 0/1
  Constant1/1 -> 00/1
  Constant2/1 -> Else Center/1(In1)
  Constant3/1 -> If Down to rest arm. UAV to hover/1(In1)
  Else Center/2(Out1) -> Merge1/2
  If Down to rest arm. UAV to hover/1(Out1) -> Merge/1

== system PWM_Test/Kinect/Subsystem1/Up or Center or Down/If Up or Center ==
  Y: RH : Inport
  Y: RSh : Inport  Port=2
  Action Port : ActionPort  ActionType=then
  Buffer : Constant  Value=0.14
  Constant : Constant  Value=0
  Constant1 : Constant  Value=0
  Constant2 : Constant
  Constant3 : Constant
  Else Center : Subsystem  TreatAsAtomicUnit=on
  If : If
  If Top : Subsystem  TreatAsAtomicUnit=on
  Merge : Merge  InitialOutput=[0]
  Merge1 : Merge  InitialOutput=[0]
  Subtract1 : Sum  Inputs=+-
  Subtract2 : Sum  Inputs=+-
  Top : Outport
  Center : Outport  Port=2
  0 : Outport  Port=3
  00 : Outport  Port=4
  wires:
  Buffer/1 -> Subtract2/2
  Subtract2/1 -> If/1
  If/1 -> If Top/Action
  If/2 -> Else Center/Action
  Y: RH/1 -> Subtract1/1
  Y: RSh/1 -> Subtract1/2
  Subtract1/1 -> Subtract2/1
  If Top/1(Out1) -> Merge/1
  Else Center/1(0) -> Merge/2
  Merge/1 -> Top/1
  Merge1/1 -> Center/1
  If Top/2(0) -> Merge1/1
  Else Center/2(Out1) -> Merge1/2
  Constant/1 -> 0/1
  Constant1/1 -> 00/1
  Constant2/1 -> If Top/1(In1)
  Constant3/1 -> Else Center/1(In1)

== system PWM_Test/Vicon_Data/Raw Quad Pose from Vicon/Process Vicon Raw Data1/Flip_pi1 ==
  Angle : Inport
  Add : Sum  Inputs=-+
  Compare To Constant1 : simulink/Logic and Bit Operations/Compare To Constant  SystemSampleTime=-1  relop=>  const=pi  LogicOutDataTypeMode=uint8  ZeroCross=off
  Constant : Constant  Value=2*pi
  Data Type Duplicate : DataTypeDuplicate
  Flip_0_to_2pi : Subsystem
      mask Type: Flip zero to 2pi
      mask Description: Flips the inputs into the range zero to +2pi
      mask Help: Flips the inputs into the range zero to +2pi
      mask Display: disp('Flip_0_2pi')
  Switch : Switch  Criteria=u2 ~= 0
  Angle_Flip : Outport
  wires:
  Angle/1 -> Flip_0_to_2pi/1(Angle), Data Type Duplicate/2
  Flip_0_to_2pi/1(Angle_Flip) -> Switch/3, Compare To Constant1/1, Add/2
  Compare To Constant1/1 -> Switch/2
  Constant/1 -> Add/1
  Add/1 -> Switch/1
  Switch/1 -> Angle_Flip/1, Data Type Duplicate/1

== system PWM_Test/Vicon_Data/Raw Quad Pose from Vicon/Process Vicon Raw Data6/Flip_pi1 ==
  Angle : Inport
  Add : Sum  Inputs=-+
  Compare To Constant1 : simulink/Logic and Bit Operations/Compare To Constant  SystemSampleTime=-1  relop=>  const=pi  LogicOutDataTypeMode=uint8  ZeroCross=off
  Constant : Constant  Value=2*pi
  Data Type Duplicate : DataTypeDuplicate
  Flip_0_to_2pi : Subsystem
      mask Type: Flip zero to 2pi
      mask Description: Flips the inputs into the range zero to +2pi
      mask Help: Flips the inputs into the range zero to +2pi
      mask Display: disp('Flip_0_2pi')
  Switch : Switch  Criteria=u2 ~= 0
  Angle_Flip : Outport
  wires:
  Angle/1 -> Flip_0_to_2pi/1(Angle), Data Type Duplicate/2
  Flip_0_to_2pi/1(Angle_Flip) -> Switch/3, Compare To Constant1/1, Add/2
  Compare To Constant1/1 -> Switch/2
  Constant/1 -> Add/1
  Add/1 -> Switch/1
  Switch/1 -> Angle_Flip/1, Data Type Duplicate/1

== system PWM_Test/Vicon_Data/Raw Quad Pose from Vicon/Process Vicon Raw Data7/Flip_pi1 ==
  Angle : Inport
  Add : Sum  Inputs=-+
  Compare To Constant1 : simulink/Logic and Bit Operations/Compare To Constant  SystemSampleTime=-1  relop=>  const=pi  LogicOutDataTypeMode=uint8  ZeroCross=off
  Constant : Constant  Value=2*pi
  Data Type Duplicate : DataTypeDuplicate
  Flip_0_to_2pi : Subsystem
      mask Type: Flip zero to 2pi
      mask Description: Flips the inputs into the range zero to +2pi
      mask Help: Flips the inputs into the range zero to +2pi
      mask Display: disp('Flip_0_2pi')
  Switch : Switch  Criteria=u2 ~= 0
  Angle_Flip : Outport
  wires:
  Switch/1 -> Data Type Duplicate/1, Angle_Flip/1
  Add/1 -> Switch/1
  Constant/1 -> Add/1
  Compare To Constant1/1 -> Switch/2
  Flip_0_to_2pi/1(Angle_Flip) -> Add/2, Compare To Constant1/1, Switch/3
  Angle/1 -> Data Type Duplicate/2, Flip_0_to_2pi/1(Angle)

== system PWM_Test/Kinect/Subsystem/Left or Center or Right/If Action Subsystem/Else Center ==
  In1 : Inport
  Action Port : ActionPort  InitializeStates=reset  ActionType=else
  Constant : Constant  Value=0
  Out1 : Outport
  0 : Outport  Port=2
  wires:
  In1/1 -> Out1/1
  Constant/1 -> 0/1

== system PWM_Test/Kinect/Subsystem/Left or Center or Right/If Action Subsystem/If Left ==
  In1 : Inport
  Action Port : ActionPort  InitializeStates=reset  ActionType=then
  Constant : Constant  Value=0
  Out1 : Outport
  0 : Outport  Port=2
  wires:
  In1/1 -> Out1/1
  Constant/1 -> 0/1

== system PWM_Test/Kinect/Subsystem/Left or Center or Right/If Action Subsystem1/Else Hover ==
  In1 : Inport
  Action Port : ActionPort  InitializeStates=reset  ActionType=else
  Abs : Abs
  Constant : Constant  Value=0
  Out1 : Outport
  0 : Outport  Port=2
  wires:
  In1/1 -> Abs/1
  Abs/1 -> Out1/1
  Constant/1 -> 0/1

== system PWM_Test/Kinect/Subsystem/Left or Center or Right/If Action Subsystem1/If Right ==
  In1 : Inport
  Action Port : ActionPort  InitializeStates=reset  ActionType=then
  Constant : Constant  Value=0
  Out1 : Outport
  0 : Outport  Port=2
  wires:
  In1/1 -> Out1/1
  Constant/1 -> 0/1

== system PWM_Test/Kinect/Subsystem/Up or Center or Down/If Down or Center/Else Center ==
  In1 : Inport
  Action Port : ActionPort  ActionType=else
  Abs : Abs
  Constant : Constant  Value=0
  0 : Outport
  Out1 : Outport  Port=2
  wires:
  In1/1 -> Abs/1
  Abs/1 -> Out1/1
  Constant/1 -> 0/1

== system PWM_Test/Kinect/Subsystem/Up or Center or Down/If Down or Center/If Down to rest arm. UAV to hover ==
  In1 : Inport
  Action Port : ActionPort  ActionType=then
  Constant : Constant  Value=0
  Out1 : Outport
  0 : Outport  Port=2
  wires:
  In1/1 -> Out1/1
  Constant/1 -> 0/1

== system PWM_Test/Kinect/Subsystem/Up or Center or Down/If Down or Center/UAV to move down ==
  In1 : Inport
  Action Port : ActionPort  ActionType=elseif
  Constant : Constant  Value=0
  Out1 : Outport
  0 : Outport  Port=2
  wires:
  In1/1 -> Out1/1
  Constant/1 -> 0/1

== system PWM_Test/Kinect/Subsystem/Up or Center or Down/If Up or Center/Else Center ==
  In1 : Inport
  Action Port : ActionPort  ActionType=else
  Abs : Abs
  Constant : Constant  Value=0
  0 : Outport
  Out1 : Outport  Port=2
  wires:
  In1/1 -> Abs/1
  Abs/1 -> Out1/1
  Constant/1 -> 0/1

== system PWM_Test/Kinect/Subsystem/Up or Center or Down/If Up or Center/If Top ==
  In1 : Inport
  Action Port : ActionPort  ActionType=then
  Constant : Constant  Value=0
  Out1 : Outport
  0 : Outport  Port=2
  wires:
  In1/1 -> Out1/1
  Constant/1 -> 0/1

== system PWM_Test/Kinect/Subsystem1/Left or Center or Right/Left or Center/Else Center ==
  In1 : Inport
  Action Port : ActionPort  InitializeStates=reset  ActionType=else
  Constant : Constant  Value=0
  Out1 : Outport
  0 : Outport  Port=2
  wires:
  In1/1 -> Out1/1
  Constant/1 -> 0/1

== system PWM_Test/Kinect/Subsystem1/Left or Center or Right/Left or Center/If Left ==
  In1 : Inport
  Action Port : ActionPort  InitializeStates=reset  ActionType=then
  Constant : Constant  Value=0
  Out1 : Outport
  0 : Outport  Port=2
  wires:
  In1/1 -> Out1/1
  Constant/1 -> 0/1

== system PWM_Test/Kinect/Subsystem1/Left or Center or Right/Right or Center/Else Center ==
  In1 : Inport
  Action Port : ActionPort  InitializeStates=reset  ActionType=else
  Abs : Abs
  Constant : Constant  Value=0
  Out1 : Outport
  0 : Outport  Port=2
  wires:
  In1/1 -> Abs/1
  Abs/1 -> Out1/1
  Constant/1 -> 0/1

== system PWM_Test/Kinect/Subsystem1/Left or Center or Right/Right or Center/If Right ==
  In1 : Inport
  Action Port : ActionPort  InitializeStates=reset  ActionType=then
  Constant : Constant  Value=0
  Out1 : Outport
  0 : Outport  Port=2
  wires:
  In1/1 -> Out1/1
  Constant/1 -> 0/1

== system PWM_Test/Kinect/Subsystem1/Up or Center or Down/If Down or Center/Else Center ==
  In1 : Inport
  Action Port : ActionPort  ActionType=else
  Abs : Abs
  Constant : Constant  Value=0
  0 : Outport
  Out1 : Outport  Port=2
  wires:
  In1/1 -> Abs/1
  Abs/1 -> Out1/1
  Constant/1 -> 0/1

== system PWM_Test/Kinect/Subsystem1/Up or Center or Down/If Down or Center/If Down to rest arm. UAV to hover ==
  In1 : Inport
  Action Port : ActionPort  ActionType=then
  Constant : Constant  Value=0
  Out1 : Outport
  0 : Outport  Port=2
  wires:
  In1/1 -> Out1/1
  Constant/1 -> 0/1

== system PWM_Test/Kinect/Subsystem1/Up or Center or Down/If Up or Center/Else Center ==
  In1 : Inport
  Action Port : ActionPort  ActionType=else
  Abs : Abs
  Constant : Constant  Value=0
  0 : Outport
  Out1 : Outport  Port=2
  wires:
  In1/1 -> Abs/1
  Abs/1 -> Out1/1
  Constant/1 -> 0/1

== system PWM_Test/Kinect/Subsystem1/Up or Center or Down/If Up or Center/If Top ==
  In1 : Inport
  Action Port : ActionPort  ActionType=then
  Constant : Constant  Value=0
  Out1 : Outport
  0 : Outport  Port=2
  wires:
  In1/1 -> Out1/1
  Constant/1 -> 0/1

== system PWM_Test/Vicon_Data/Raw Quad Pose from Vicon/Process Vicon Raw Data1/Flip_pi1/Flip_0_to_2pi ==
  Angle : Inport
  Add : Sum
  Compare To Constant1 : simulink/Logic and Bit Operations/Compare To Constant  SystemSampleTime=-1  relop=<  const=0  LogicOutDataTypeMode=uint8  ZeroCross=off
  Constant : Constant  Value=2*pi
  Data Type Duplicate : DataTypeDuplicate
  Flip_2pi : Subsystem
      mask Type: Flip -2pi to 2pi
      mask Description: Flips the inputs into the range -2pi to +2pi
      mask Help: Flips the inputs into the range -2pi to +2pi
      mask Display: disp('Flip_2pi')
  Switch : Switch  Criteria=u2 ~= 0
  Angle_Flip : Outport
  wires:
  Flip_2pi/1(Angle_Flip) -> Compare To Constant1/1, Add/2, Switch/3
  Compare To Constant1/1 -> Switch/2
  Constant/1 -> Add/1
  Add/1 -> Switch/1
  Angle/1 -> Flip_2pi/1(Angle), Data Type Duplicate/2
  Switch/1 -> Angle_Flip/1, Data Type Duplicate/1

== system PWM_Test/Vicon_Data/Raw Quad Pose from Vicon/Process Vicon Raw Data6/Flip_pi1/Flip_0_to_2pi ==
  Angle : Inport
  Add : Sum
  Compare To Constant1 : simulink/Logic and Bit Operations/Compare To Constant  SystemSampleTime=-1  relop=<  const=0  LogicOutDataTypeMode=uint8  ZeroCross=off
  Constant : Constant  Value=2*pi
  Data Type Duplicate : DataTypeDuplicate
  Flip_2pi : Subsystem
      mask Type: Flip -2pi to 2pi
      mask Description: Flips the inputs into the range -2pi to +2pi
      mask Help: Flips the inputs into the range -2pi to +2pi
      mask Display: disp('Flip_2pi')
  Switch : Switch  Criteria=u2 ~= 0
  Angle_Flip : Outport
  wires:
  Flip_2pi/1(Angle_Flip) -> Compare To Constant1/1, Add/2, Switch/3
  Compare To Constant1/1 -> Switch/2
  Constant/1 -> Add/1
  Add/1 -> Switch/1
  Angle/1 -> Flip_2pi/1(Angle), Data Type Duplicate/2
  Switch/1 -> Angle_Flip/1, Data Type Duplicate/1

== system PWM_Test/Vicon_Data/Raw Quad Pose from Vicon/Process Vicon Raw Data7/Flip_pi1/Flip_0_to_2pi ==
  Angle : Inport
  Add : Sum
  Compare To Constant1 : simulink/Logic and Bit Operations/Compare To Constant  SystemSampleTime=-1  relop=<  const=0  LogicOutDataTypeMode=uint8  ZeroCross=off
  Constant : Constant  Value=2*pi
  Data Type Duplicate : DataTypeDuplicate
  Flip_2pi : Subsystem
      mask Type: Flip -2pi to 2pi
      mask Description: Flips the inputs into the range -2pi to +2pi
      mask Help: Flips the inputs into the range -2pi to +2pi
      mask Display: disp('Flip_2pi')
  Switch : Switch  Criteria=u2 ~= 0
  Angle_Flip : Outport
  wires:
  Switch/1 -> Data Type Duplicate/1, Angle_Flip/1
  Angle/1 -> Data Type Duplicate/2, Flip_2pi/1(Angle)
  Add/1 -> Switch/1
  Constant/1 -> Add/1
  Compare To Constant1/1 -> Switch/2
  Flip_2pi/1(Angle_Flip) -> Switch/3, Add/2, Compare To Constant1/1

== system PWM_Test/Vicon_Data/Raw Quad Pose from Vicon/Process Vicon Raw Data1/Flip_pi1/Flip_0_to_2pi/Flip_2pi ==
  Angle : Inport
  Bias : Bias  Bias=-2*pi
  Constant : Constant  Value=2*pi
  Data Type Duplicate : DataTypeDuplicate
  Modulo : Math  Operator=mod  SaturateOnIntegerOverflow=on
  Sign1 : Signum
  Switch : Switch
  Angle_Flip : Outport
  wires:
  Angle/1 -> Modulo/1, Sign1/1, Data Type Duplicate/1
  Constant/1 -> Modulo/2
  Modulo/1 -> Bias/1, Switch/1
  Sign1/1 -> Switch/2
  Bias/1 -> Switch/3
  Switch/1 -> Angle_Flip/1, Data Type Duplicate/2

== system PWM_Test/Vicon_Data/Raw Quad Pose from Vicon/Process Vicon Raw Data6/Flip_pi1/Flip_0_to_2pi/Flip_2pi ==
  Angle : Inport
  Bias : Bias  Bias=-2*pi
  Constant : Constant  Value=2*pi
  Data Type Duplicate : DataTypeDuplicate
  Modulo : Math  Operator=mod  SaturateOnIntegerOverflow=on
  Sign1 : Signum
  Switch : Switch
  Angle_Flip : Outport
  wires:
  Angle/1 -> Modulo/1, Sign1/1, Data Type Duplicate/1
  Constant/1 -> Modulo/2
  Modulo/1 -> Bias/1, Switch/1
  Sign1/1 -> Switch/2
  Bias/1 -> Switch/3
  Switch/1 -> Angle_Flip/1, Data Type Duplicate/2

== system PWM_Test/Vicon_Data/Raw Quad Pose from Vicon/Process Vicon Raw Data7/Flip_pi1/Flip_0_to_2pi/Flip_2pi ==
  Angle : Inport
  Bias : Bias  Bias=-2*pi
  Constant : Constant  Value=2*pi
  Data Type Duplicate : DataTypeDuplicate
  Modulo : Math  Operator=mod  SaturateOnIntegerOverflow=on
  Sign1 : Signum
  Switch : Switch
  Angle_Flip : Outport
  wires:
  Switch/1 -> Data Type Duplicate/2, Angle_Flip/1
  Bias/1 -> Switch/3
  Sign1/1 -> Switch/2
  Modulo/1 -> Switch/1, Bias/1
  Constant/1 -> Modulo/2
  Angle/1 -> Data Type Duplicate/1, Sign1/1, Modulo/1

== matlab function Planning/Yaw Controller/MATLAB Function ==
  data: u input double; y output double
function y = fcn(u)
%#codegen
y = u;
if y > pi    
    y = y - 2*pi;
elseif y < -pi
        y = y + 2*pi;
end

== stateflow chart Planning/Trajectory Logic/UAV SF ==
  state AirBorne
    state TakeOff
      du:HoverThrottle = (H0 - HoverThrottle)*3*DeltaT + HoverThrottle ;
    state PWM900
      en:
      PWM=900;
    state PWM1600
      en:
      PWM=1600;
    (default) -> TakeOff : {PosDesired = Pos;  PosDesired[2] =-1.2;}
    TakeOff -> PWM1600 [order 2] : [RC[5] > 0.5]
    TakeOff -> PWM900 [order 1] : [RC[5] > 0.5]
  state Landing
    state Descending
      en:PosDesired = Pos;
      du:PosDesired[2] = (0.1- PosDesired[2])*1*DeltaT + PosDesired[2] ;
    state CutThrottle
      en: PWM=1600;
      du:HoverThrottle = (0.0- HoverThrottle)*3*DeltaT + HoverThrottle ;
    (default) -> Descending
    Descending -> CutThrottle : [Pos[2] >(0.0 -0.1)]
  Landing -> AirBorne : [RC[6] > 0.5]
  AirBorne -> Landing : [RC[6] < -0.5]
  (default) -> Landing : {HoverThrottle = 0;}
  data: PosDesired output double size=4; HoverThrottle output double size=1; Mode output uint8 size=1; RC input double size=8; Pos input double size=4; PerchPos input double size=4; DeltaT parameter double size=1; H0 parameter double size=1; Kl parameter double size=1; VelCmd local double size=2 =0; PWM output double; PerchError input double; PI parameter double size=1; draw input double size=3; descentrate local double; LeftHand input double; KinectTracking input double; UpDown local double; FrontBack local double; LeftRight local double; LXcounter local double; LYcounter local double; LZcounter local double; XYZchecker local double; RightHand input double; Rcounter local double; ClawStatus local double; LHRH local double; Rotation local double
